simulink model "Gravity_Compensate"  (R2018b)
settings: Solver=FixedStepAuto  StartTime=0.0  StopTime=inf  FixedStep=0.001  RelTol=1e-3  EnableMultiTasking=on
values from neighbouring files (symbols this model uses):
  Dis_Coff = [0.42361 0.19319 -26.689 1.2064 -2.9972 4045.7 -3.3883 3.6846 291430]    [Robot_Parameters_Ident_With_Disturbance.mat]
  F1G = 0.2    [Main_Code.m]    (also in Main_Code_Gravity_Compensation.m)
  F2G = 0.2    [Main_Code.m]    (also in Main_Code_Gravity_Compensation.m)
  F3G = 0.005    [Main_Code.m]    (also in Main_Code_Gravity_Compensation.m)
  phi_Dynamic = [phi0;phi1;phi2;phi3;phi4;phi5;phi6;phi7]    [Parameters_Builder.m]    (also in Robot_Parameters.mat = [0.73163251 -0.0393 0 2.40643096032e-18 0.000785329049449 0.; Robot_Parameters_Ident.mat = [0.78122 -0.0393 0 2.40643096032e-18 0.000785329049449 0.000; Robot_Parameters_Ident_With_Disturbance.mat = [0.78122 -0.0393 0 2.40643096032e-18 0.000785329049449 0.000)
  phi_Kinematic = [l__0;l__1;l__3;l__5;l__2;l__7;theta;alpha;d__0;l__x35;l__z35;psi0]    [Parameters_Builder.m]    (also in Robot_Parameters.mat = [0.006 0.182 0.05 0.115 0.07 0.0342 0.733038285838 0.8726646; Robot_Parameters_Ident.mat = [0.006 0.182 0.05 0.115 0.07 0.0342 0.733038285838 0.8726646; Robot_Parameters_Ident_With_Disturbance.mat = [0.006 0.182 0.05 0.115 0.07 0.0342 0.733038285838 0.8726646)
libraries: neural x94, xpcrtudplib x3, xpcutilitieslib x2, slrtlib x1
(part 3 of 3)

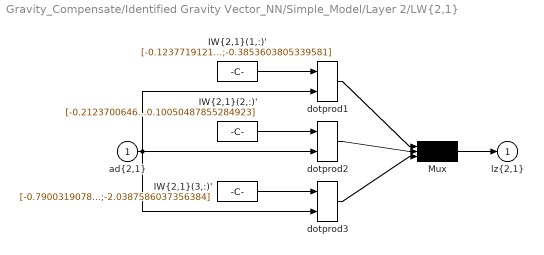
== system Gravity_Compensate/Identified Gravity Vector_NN/Simple_Model/Layer 2/LW{2,1} ==
  "ad{2,1}" : Inport  PortDimensions=40
      mask Display: e = 0.06;c1 = [120 230 180]/255;c2 = ([120 230 180]+0)/(256+128);c3 = ([120 230 180]+128)/(256+128);patch([0 1 1 0],[0 0 1 1],c1);patch([0 1 1 1-e 1-e 0+e],[0 0 1 1-e 0+e 0+e],c2);patch([0 0 1 1-e 0+e 0+e],[0 1 1 1-e 1-e 0+e],c3);plot([0 1 1 0 0],[0 0 1 1 0]);
  "IW{2,1}(1,:)'" : Constant  Value=[-0.12377191211538843;0.47986142990758968;0.071466232965383902;-0.014643661998884991;-0.036348558938390195;-1.2683784142329346;0.048710591521782094;-0.15588565925443046;-0.29593921510480592;0.83254224929096454;0.095433439724007182;0.23086701536801224;0.015407278077396039;0.18634370336900394;-0.10644950816853133;-0.8890739968674527;0.095646401259416938;-0.22362466624332347;-0.081295963255982803;0.22073406075035309;0.3832484095539625;-0.33181408968776566;-0.4512826684512522;-0.75353013394929214;-0.13480679804397866;0.47431684665500434;0.23360844504165507;0.34355041450051022;-0.44737259560248294;-0.60005340860707446;0.11557813742975434;-0.55696851655690749;-0.57362258340574612;0.38585851480907596;-0.22383283008524452;1.0361330561174151;-0.5058986808767082;0.25656685245000227;0.23364293488333043;-0.3853603805339581]
      mask Display: e = 0.06;c1 = [120 150 230]/255;c2 = ([120 150 230]+0)/383;c3 = ([120 150 230]+128)/383;patch([0 1 1 0],[0 0 1 1],c1);patch([0 1 1 1-e 1-e 0+e],[0 0 1 1-e 0+e 0+e],c2);patch([0 0 1 1-e 0+e 0+e],[0 1 1 1-e 1-e 0+e],c3);plot([0 1 1 0 0],[0 0 1 1 0]);disp('weights');
  "IW{2,1}(2,:)'" : Constant  Value=[-0.21237006469585565;0.38972766835962391;0.061338232745156138;-0.59670701416894945;0.041883594878444855;0.50115597302835624;-0.063274397097907539;-0.21976598408006989;-0.56658233119011836;0.27089627097339691;0.11589549004923319;-0.37350037412217291;0.85866725683274836;0.04964911563044213;-0.31998149737348414;0.41597937966006465;0.13855157386504593;0.12735246667736255;0.28364329190194987;0.12816907808314534;-0.061868161448917075;0.069281366199724692;-0.91585359020242696;0.72648071784342494;-0.34425899670118615;0.33596403308110079;0.20344250869877367;-0.20372062860536683;0.33918366194568678;0.042008389697913651;-0.14291313373246031;0.43898446034834443;0.38229905245172285;0.46078224913163723;-0.83072723510083857;0.1083489828094826;-0.055965093481781386;0.33114948189972926;0.17304160737736651;0.10050487855284923]
      mask Display: e = 0.06;c1 = [120 150 230]/255;c2 = ([120 150 230]+0)/383;c3 = ([120 150 230]+128)/383;patch([0 1 1 0],[0 0 1 1],c1);patch([0 1 1 1-e 1-e 0+e],[0 0 1 1-e 0+e 0+e],c2);patch([0 0 1 1-e 0+e 0+e],[0 1 1 1-e 1-e 0+e],c3);plot([0 1 1 0 0],[0 0 1 1 0]);disp('weights');
  "IW{2,1}(3,:)'" : Constant  Value=[-0.79003190788975919;1.6908270976961295;1.2494452149393176;2.1032315733142686;-4.3563090718320989;-1.2576689893497666;1.489416888303124;-1.025094213956429;-1.5816571501161376;-1.8299202207716927;3.3069713643104919;1.3834371081180556;0.50320865825156125;1.7106126090243972;-2.7405949722191192;6.7140525799211321;-0.74302022863882122;-1.1622803010305198;-1.4453375973251941;-0.77446014496877136;0.74560705664111704;-1.0783910048420244;1.0551652987829556;-0.52378061703590328;0.83301878392234019;-0.92348331624611746;-1.1500644949566845;1.7331740221827683;-2.6338572860317702;1.6680942325252988;-1.2699279852658185;0.79474895214471586;-0.28757949719638143;-0.3920215418354962;1.5883940929987677;-1.7437223965027382;-0.4941004380187739;-3.303144701318562;-1.2416985014096205;-2.0387586037356384]
      mask Display: e = 0.06;c1 = [120 150 230]/255;c2 = ([120 150 230]+0)/383;c3 = ([120 150 230]+128)/383;patch([0 1 1 0],[0 0 1 1],c1);patch([0 1 1 1-e 1-e 0+e],[0 0 1 1-e 0+e 0+e],c2);patch([0 0 1 1-e 0+e 0+e],[0 1 1 1-e 1-e 0+e],c3);plot([0 1 1 0 0],[0 0 1 1 0]);disp('weights');
  Mux : Mux  Inputs=3
      mask Display: e = 0.06;c1 = [120 150 230]/255;c2 = ([120 150 230]+0)/383;c3 = ([120 150 230]+128)/383;patch([0 1 1 0],[0 0 1 1],c1);patch([0 1 1 1-e 1-e 0+e],[0 0 1 1-e 0+e 0+e],c2);patch([0 0 1 1-e 0+e 0+e],[0 1 1 1-e 1-e 0+e],c3);plot([0 1 1 0 0],[0 0 1 1 0]);disp('Mux');
  dotprod1 : neural/Weight Functions/dotprod
  dotprod2 : neural/Weight Functions/dotprod
  dotprod3 : neural/Weight Functions/dotprod
  "lz{2,1}" : Outport
      mask Display: e = 0.06;c1 = [120 230 180]/255;c2 = ([120 230 180]+0)/(256+128);c3 = ([120 230 180]+128)/(256+128);patch([0 1 1 0],[0 0 1 1],c1);patch([0 1 1 1-e 1-e 0+e],[0 0 1 1-e 0+e 0+e],c2);patch([0 0 1 1-e 0+e 0+e],[0 1 1 1-e 1-e 0+e],c3);plot([0 1 1 0 0],[0 0 1 1 0]);
  wires:
  "IW{2,1}(1,:)'"/1 -> dotprod1/1
  "ad{2,1}"/1 -> dotprod1/2, dotprod2/2, dotprod3/2
  dotprod1/1 -> Mux/1
  "IW{2,1}(2,:)'"/1 -> dotprod2/1
  dotprod2/1 -> Mux/2
  "IW{2,1}(3,:)'"/1 -> dotprod3/1
  dotprod3/1 -> Mux/3
  Mux/1 -> "lz{2,1}"/1

== matlab function Gravity_Compensate/Gravity_Friction_Disturbance/Subsystem6/MATLAB Function1 ==
  data: q input; G output; phi_Kinematic input; phi_Dynamic input
function G = fcn(q,phi_Kinematic,phi_Dynamic)

G = G_Vector(q,phi_Kinematic,phi_Dynamic);

end

== matlab function Gravity_Compensate/Gravity_Friction_Disturbance/Jacobian ==
  data: q input; Tau output; phi_Kinematic input; Dis_Coff input
function Tau = fcn(q,phi_Kinematic,Dis_Coff)

phi=q(1);
psi=q(2);
d=q(3);

l__0=phi_Kinematic(1);
l__1=phi_Kinematic(2);
l__3=phi_Kinematic(3);
l__5=phi_Kinematic(4);
l__2=phi_Kinematic(5);
l__7=phi_Kinematic(6);
theta=phi_Kinematic(7);
alpha=phi_Kinematic(8);
d__0=phi_Kinematic(9);
l__x35=phi_Kinematic(10);
l__z35=phi_Kinematic(11);

%% 

a1=Dis_Coff(1:3,1);
a2=Dis_Coff(4:6,1);
a3=Dis_Coff(7:9,1);



beta=alpha;
    J=[-cos(theta) * sin(phi) * sin(psi + beta) * d -sin(theta) * sin(psi + beta) * d + cos(theta) * cos(phi) * cos(psi + beta) * d sin(theta) * cos(psi + beta) + cos(theta) * cos(phi) * sin(psi + beta); cos(phi) * sin(psi + beta) * d sin(phi) * cos(psi + beta) * d sin(phi) * sin(psi + beta); sin(theta) * sin(phi) * sin(psi + beta) * d -sin(psi + beta) * cos(theta) * d - sin(theta) * cos(phi) * cos(psi + beta) * d cos(theta) * cos(psi + beta) - sin(theta) * cos(phi) * sin(psi + beta);];
    F_ext=diag(a1)*q+diag(a2)*q.^2+diag(a3)*q.^3;
    Tau   =  J'*F_ext;
    
    
end
